simulink model "ANN_MLP_BP_Incremental_Mode_Training"  (Simulink 6.0)
settings: Solver=FixedStepDiscrete  StartTime=0.0  StopTime=10000  RelTol=1e-3
undefined symbols (not defined in the file): magnitude
libraries: simulink x10
settings Model: Creator=marcelo  LastModifiedBy=Marcelo
settings HardwareCC: TargetHWDeviceType=32-bit Generic

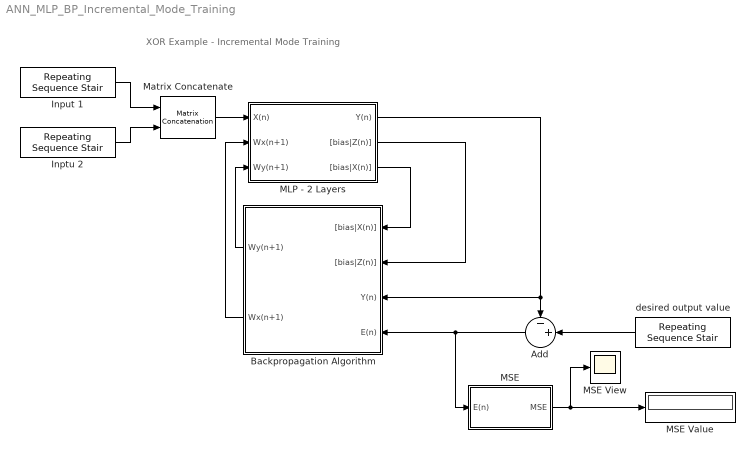
== system ANN_MLP_BP_Incremental_Mode_Training ==
  note: XOR Example - Incremental Mode Training
  Add : Sum  Orientation=left  Inputs=-+|  OutDataType=fixdt(1,16,0)  OutScaling=[]
  Backpropagation Algorithm : Subsystem  Orientation=left  mask(Backpropagation Algorithm){mu=0.2, alpha=0.001, N=1, p=2, H=4, m=1}
      mask prompts: N "training size:"; p "Number of the inputs:"; H "Number of hidden neurons:"; m "Number of output neurons:"
      mask help:
      | Backpropagation Algorithm
      |
      | Prof. Marcelo A. C. Fernandes
      | DCA - CT - UFRN
      | mfernandes@dca.ufrn.br
      mask Help:
      | Backpropagation Algorithm
      | 
      | Prof. Marcelo A. C. Fernandes
      | DCA - CT - UFRN
      | mfernandes@dca.ufrn.br
  Inptu 2 : simulink/Sources/Repeating Sequence Stair  OutValues=[0 1 0 1]  tsamp=1  OutputDataTypeScalingMode=Specify via dialog  OutDataType=float('double')  ConRadixGroup=Best Precision: Vector-wise  OutScaling=2^-12
  Input 1 : simulink/Sources/Repeating Sequence Stair  OutValues=[0 0 1 1]  tsamp=1  OutputDataTypeScalingMode=Specify via dialog  OutDataType=float('double')  ConRadixGroup=Best Precision: Vector-wise  OutScaling=2^-12
  MLP - 2 Layers : Subsystem  mask(Multilayer Perceptron (MLP) - 2 Layers){N=1, valorLimiar=-1, p=2, H=4, m=1}
      mask prompts: N "training size:"; valorLimiar "Bias value:"; p "Number of the inputs:"; H "Number of hidden neurons:"; m "Number of output neurons:"
      mask help:
      | Multilayer Perceptron (MLP) - 2 Layers
      |
      | Prof. Marcelo Augusto Costa Fernandes
      | DCA - CT - UFRN
      | mfernandes@dca.ufrn.br
      mask Help:
      | Multilayer Perceptron (MLP) - 2 Layers
      | 
      | Prof. Marcelo Augusto Costa Fernandes
      | DCA - CT - UFRN
      | mfernandes@dca.ufrn.br
  MSE : Subsystem  mask(MSE){N=1, m=1}
      mask prompts: N "training size:"; m "Number of output neurons:"
      mask help:
      | MSE
      |
      | Prof. Marcelo Augusto Costa Fernandes
      | DCA - CT - UFRN
      | mfernandes@dca.ufrn.br
      mask Help:
      | MSE
      | 
      | Prof. Marcelo Augusto Costa Fernandes
      | DCA - CT - UFRN
      | mfernandes@dca.ufrn.br
  MSE Value : Display
  MSE View : Scope
      settings: MaxDataPoints=5000000
  Matrix Concatenate : simulink/Math Operations/Matrix Concatenation  numInports=2  catMethod=Vertical
  desired output value : simulink/Sources/Repeating Sequence Stair  Orientation=left  OutValues=[0 1 1 0]  tsamp=1  OutputDataTypeScalingMode=Specify via dialog  OutDataType=float('double')  ConRadixGroup=Best Precision: Vector-wise  OutScaling=2^-12
  wires:
  Add/1 -> Backpropagation Algorithm/4(E(n)), MSE/1(E(n))
  MLP - 2 Layers/2("[bias|Z(n)]") -> Backpropagation Algorithm/2("[bias|Z(n)]")
  Backpropagation Algorithm/2(Wx(n+1)) -> MLP - 2 Layers/2(Wx(n+1))
  Backpropagation Algorithm/1(Wy(n+1)) -> MLP - 2 Layers/3(Wy(n+1))
  MLP - 2 Layers/3("[bias|X(n)]") -> Backpropagation Algorithm/1("[bias|X(n)]")
  Input 1/1 -> Matrix Concatenate/1
  Inptu 2/1 -> Matrix Concatenate/2
  MLP - 2 Layers/1(Y(n)) -> Add/1, Backpropagation Algorithm/3(Y(n))
  Matrix Concatenate/1 -> MLP - 2 Layers/1(X(n))
  desired output value/1 -> Add/2
  MSE/1(MSE) -> MSE Value/1, MSE View/1

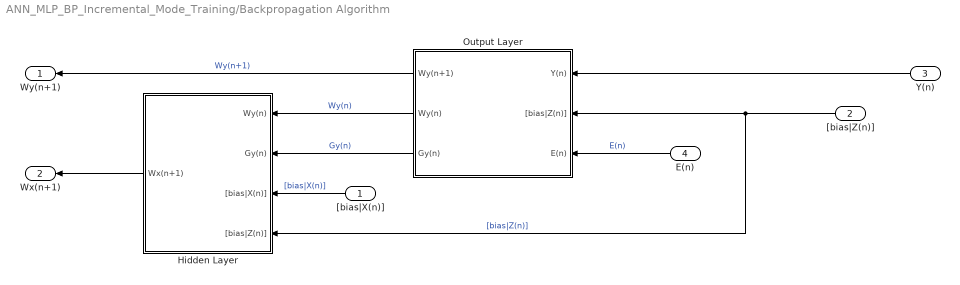
== system ANN_MLP_BP_Incremental_Mode_Training/Backpropagation Algorithm ==
  "[bias|X(n)]" : Inport  Orientation=left  Port=1  OutDataType=fixdt(1,16,0)  OutScaling=[]  LatchInput=off
  "[bias|Z(n)]" : Inport  Orientation=left  Port=2  OutDataType=fixdt(1,16,0)  OutScaling=[]  LatchInput=off
  Y(n) : Inport  Orientation=left  Port=3  OutDataType=fixdt(1,16,0)  OutScaling=[]  LatchInput=off
  E(n) : Inport  Orientation=left  Port=4  OutDataType=fixdt(1,16,0)  OutScaling=[]  LatchInput=off
  Hidden Layer : Subsystem  Orientation=left
  Output Layer : Subsystem  Orientation=left
  Wy(n+1) : Outport  Orientation=left  OutDataType=fixdt(1,16,0)  OutScaling=[]
  Wx(n+1) : Outport  Orientation=left  Port=2  OutDataType=fixdt(1,16,0)  OutScaling=[]
  wires:
  Output Layer/1(Wy(n+1)) -> Wy(n+1)/1  "Wy(n+1)"
  "[bias|Z(n)]"/1 -> Output Layer/2("[bias|Z(n)]"), Hidden Layer/4("[bias|Z(n)]")  "[bias|Z(n)]"
  E(n)/1 -> Output Layer/3(E(n))  "E(n)"
  Output Layer/2(Wy(n)) -> Hidden Layer/1(Wy(n))  "Wy(n)"
  Output Layer/3(Gy(n)) -> Hidden Layer/2(Gy(n))  "Gy(n)"
  "[bias|X(n)]"/1 -> Hidden Layer/3("[bias|X(n)]")  "[bias|X(n)]"
  Hidden Layer/1(Wx(n+1)) -> Wx(n+1)/1
  Y(n)/1 -> Output Layer/1(Y(n))

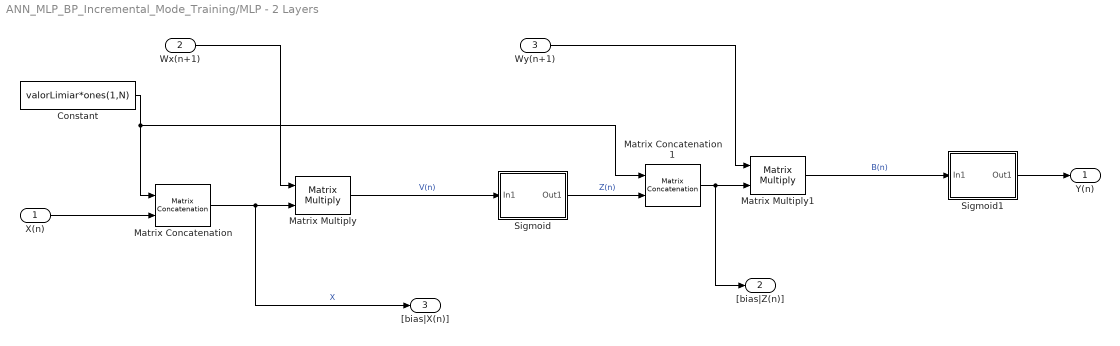
== system ANN_MLP_BP_Incremental_Mode_Training/MLP - 2 Layers ==
  X(n) : Inport  Port=1  OutDataType=fixdt(1,16,0)  OutScaling=[]  LatchInput=off
  Wx(n+1) : Inport  Port=2  OutDataType=fixdt(1,16,0)  OutScaling=[]  LatchInput=off
  Wy(n+1) : Inport  Port=3  OutDataType=fixdt(1,16,0)  OutScaling=[]  LatchInput=off
  Constant : Constant  Value=valorLimiar*ones(1,N)  VectorParams1D=off  OutDataType=fixdt(1,16,0)  OutScaling=[]
  Matrix Concatenation : simulink/Math Operations/Matrix Concatenation  numInports=2  catMethod=Vertical
  Matrix Concatenation1 : simulink/Math Operations/Matrix Concatenation  numInports=2  catMethod=Vertical
  Matrix Multiply : Product  Multiplication=Matrix(*)  OutDataType=fixdt(1,16,0)  OutScaling=[]
  Matrix Multiply1 : Product  Multiplication=Matrix(*)  OutDataType=fixdt(1,16,0)  OutScaling=[]
  Sigmoid : Subsystem
      mask Type: Sigmoid Function
      mask Description:
      | Sigmoid Function.
      | 
      | 1/(1+exp(-x))
      | 
      | Prof. Marcelo Fernandes
      | DCA - CT - UFRN
      | mfernandes@dca.ufrn.br
      mask Help:
      | Sigmoid Function.
      | 
      | 1/(1+exp(-x))
      | 
      | Prof. Marcelo Fernandes
      | DCA - CT - UFRN
      | mfernandes@dca.ufrn.br
      mask Display: plot([-8:.1:8],(1-exp(-1*[-8:.1:8]))./(1+exp(-1*[-8:.1:8])))
  Sigmoid1 : Subsystem
      mask Type: Sigmoid Function
      mask Description:
      | Sigmoid Function.
      | 
      | 1/(1+exp(-x))
      | 
      | Prof. Marcelo Fernandes
      | DCA - CT - UFRN
      | mfernandes@dca.ufrn.br
      mask Help:
      | Sigmoid Function.
      | 
      | 1/(1+exp(-x))
      | 
      | Prof. Marcelo Fernandes
      | DCA - CT - UFRN
      | mfernandes@dca.ufrn.br
      mask Display: plot([-8:.1:8],(1-exp(-1*[-8:.1:8]))./(1+exp(-1*[-8:.1:8])))
  Y(n) : Outport  OutDataType=fixdt(1,16,0)  OutScaling=[]
  "[bias|Z(n)]" : Outport  Port=2  OutDataType=fixdt(1,16,0)  OutScaling=[]
  "[bias|X(n)]" : Outport  Port=3  OutDataType=fixdt(1,16,0)  OutScaling=[]
  wires:
  Constant/1 -> Matrix Concatenation/1, Matrix Concatenation1/1
  Matrix Concatenation/1 -> Matrix Multiply/2, "[bias|X(n)]"/1  "X"
  Matrix Multiply/1 -> Sigmoid/1(In1)  "V(n)"
  X(n)/1 -> Matrix Concatenation/2
  Wx(n+1)/1 -> Matrix Multiply/1
  Matrix Multiply1/1 -> Sigmoid1/1(In1)  "B(n)"
  Sigmoid/1(Out1) -> Matrix Concatenation1/2  "Z(n)"
  Matrix Concatenation1/1 -> Matrix Multiply1/2, "[bias|Z(n)]"/1
  Wy(n+1)/1 -> Matrix Multiply1/1
  Sigmoid1/1(Out1) -> Y(n)/1

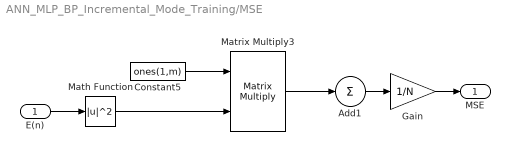
== system ANN_MLP_BP_Incremental_Mode_Training/MSE ==
  E(n) : Inport  Port=1  LatchInput=off
  Add1 : Sum  Inputs=1  OutDataType=fixdt(1,16,0)  OutScaling=[]
  Constant5 : Constant  Value=ones(1,m)  VectorParams1D=off  OutDataType=fixdt(1,16,0)  OutScaling=[]
  Gain : Gain  Gain=1/N  ParameterDataType=fixdt(1,16,0)  ParameterScaling=[]  OutDataType=fixdt(1,16,0)  OutScaling=[]
  Math Function : Math  Operator=magnitude^2  OutDataType=fixdt(1,16,0)  OutScaling=[]  SaturateOnIntegerOverflow=on
  Matrix Multiply3 : Product  Multiplication=Matrix(*)  OutDataType=fixdt(1,16,0)  OutScaling=[]
  MSE : Outport
  wires:
  Add1/1 -> Gain/1
  Constant5/1 -> Matrix Multiply3/1
  Math Function/1 -> Matrix Multiply3/2
  Matrix Multiply3/1 -> Add1/1
  E(n)/1 -> Math Function/1
  Gain/1 -> MSE/1

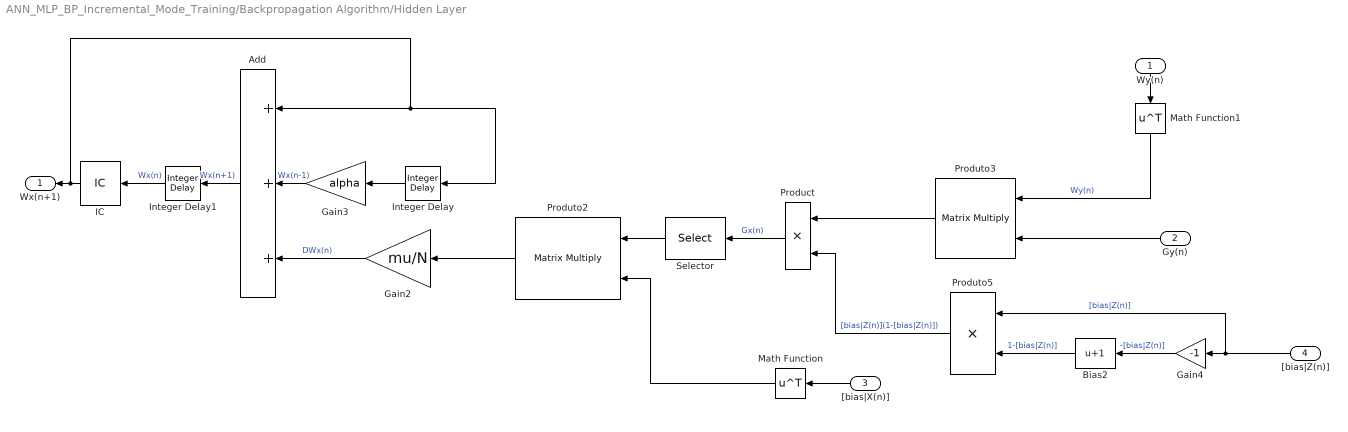
== system ANN_MLP_BP_Incremental_Mode_Training/Backpropagation Algorithm/Hidden Layer ==
  Wy(n) : Inport  Orientation=down  Port=1  OutDataType=fixdt(1,16,0)  OutScaling=[]  LatchInput=off
  Gy(n) : Inport  Orientation=left  Port=2  OutDataType=fixdt(1,16,0)  OutScaling=[]  LatchInput=off
  "[bias|X(n)]" : Inport  Orientation=left  Port=3  OutDataType=fixdt(1,16,0)  OutScaling=[]  LatchInput=off
  "[bias|Z(n)]" : Inport  Orientation=left  Port=4  OutDataType=fixdt(1,16,0)  OutScaling=[]  LatchInput=off
  Add : Sum  Orientation=left  Inputs=+++  OutDataType=fixdt(1,16,0)  OutScaling=[]
  Bias2 : Bias  Orientation=left  Bias=1
  Gain2 : Gain  Orientation=left  Gain=mu/N  ParameterDataType=fixdt(1,16,0)  ParameterScaling=[]  OutDataType=fixdt(1,16,0)  OutScaling=[]
  Gain3 : Gain  Orientation=left  Gain=alpha  ParameterDataType=fixdt(1,16,0)  ParameterScaling=[]  OutDataType=fixdt(1,16,0)  OutScaling=[]
  Gain4 : Gain  Orientation=left  Gain=-1  ParameterDataType=fixdt(1,16,0)  ParameterScaling=[]  OutDataType=fixdt(1,16,0)  OutScaling=[]
  IC : InitialCondition  Orientation=left  Value=rand(H,p+1)
  Integer Delay : simulink/Discrete/Integer Delay  Orientation=left  vinit=0.0  samptime=-1  NumDelays=1
  Integer Delay1 : simulink/Discrete/Integer Delay  Orientation=left  vinit=0.0  samptime=-1  NumDelays=1
  Math Function : Math  Orientation=left  Operator=transpose  OutDataType=fixdt(1,16,0)  OutScaling=[]  SaturateOnIntegerOverflow=on
  Math Function1 : Math  Orientation=down  Operator=transpose  OutDataType=fixdt(1,16,0)  OutScaling=[]  SaturateOnIntegerOverflow=on
  Product : Product  Orientation=left  RndMeth=Zero
  Produto2 : Product  Orientation=left  Inputs=**  Multiplication=Matrix(*)  OutDataType=fixdt(1,16,0)  OutScaling=[]
  Produto3 : Product  Orientation=left  Inputs=**  Multiplication=Matrix(*)  OutDataType=fixdt(1,16,0)  OutScaling=[]
  Produto5 : Product  Orientation=left  Inputs=**  OutDataType=fixdt(1,16,0)  OutScaling=[]
  Selector : Selector  Orientation=left  InputType=Matrix  Rows=[2:H+1]  Columns=-1  InputPortWidth=3
  Wx(n+1) : Outport  Orientation=left  OutDataType=fixdt(1,16,0)  OutScaling=[]
  wires:
  Math Function1/1 -> Produto3/1  "Wy(n)"
  Produto3/1 -> Product/1
  Wy(n)/1 -> Math Function1/1
  Gy(n)/1 -> Produto3/2
  "[bias|X(n)]"/1 -> Math Function/1
  "[bias|Z(n)]"/1 -> Produto5/1, Gain4/1  "[bias|Z(n)]"
  Gain4/1 -> Bias2/1  "-[bias|Z(n)]"
  Bias2/1 -> Produto5/2  "1-[bias|Z(n)]"
  Produto5/1 -> Product/2  "[bias|Z(n)](1-[bias|Z(n)])"
  Product/1 -> Selector/1  "Gx(n)"
  Math Function/1 -> Produto2/2
  Selector/1 -> Produto2/1
  Gain2/1 -> Add/3  "DWx(n)"
  Integer Delay/1 -> Gain3/1
  Gain3/1 -> Add/2  "Wx(n-1)"
  Produto2/1 -> Gain2/1
  Add/1 -> Integer Delay1/1  "Wx(n+1)"
  Integer Delay1/1 -> IC/1  "Wx(n)"
  IC/1 -> Wx(n+1)/1, Add/1, Integer Delay/1

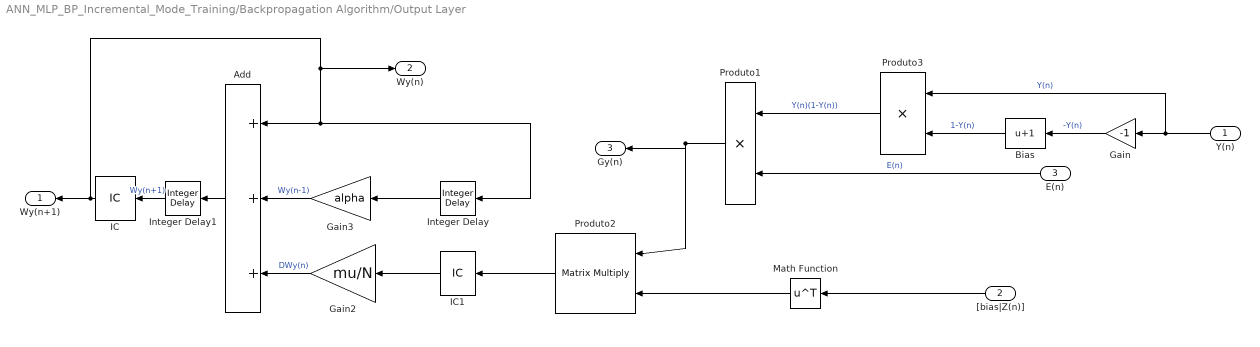
== system ANN_MLP_BP_Incremental_Mode_Training/Backpropagation Algorithm/Output Layer ==
  Y(n) : Inport  Orientation=left  Port=1  OutDataType=fixdt(1,16,0)  OutScaling=[]  LatchInput=off
  "[bias|Z(n)]" : Inport  Orientation=left  Port=2  OutDataType=fixdt(1,16,0)  OutScaling=[]  LatchInput=off
  E(n) : Inport  Orientation=left  Port=3  OutDataType=fixdt(1,16,0)  OutScaling=[]  LatchInput=off
  Add : Sum  Orientation=left  Inputs=+++  OutDataType=fixdt(1,16,0)  OutScaling=[]
  Bias : Bias  Orientation=left  Bias=1
  Gain : Gain  Orientation=left  Gain=-1  ParameterDataType=fixdt(1,16,0)  ParameterScaling=[]  OutDataType=fixdt(1,16,0)  OutScaling=[]
  Gain2 : Gain  Orientation=left  Gain=mu/N  ParameterDataType=fixdt(1,16,0)  ParameterScaling=[]  OutDataType=fixdt(1,16,0)  OutScaling=[]
  Gain3 : Gain  Orientation=left  Gain=alpha  ParameterDataType=fixdt(1,16,0)  ParameterScaling=[]  OutDataType=fixdt(1,16,0)  OutScaling=[]
  IC : InitialCondition  Orientation=left  Value=rand(m,H+1)
  IC1 : InitialCondition  Orientation=left  Value=rand(m,H+1)
  Integer Delay : simulink/Discrete/Integer Delay  Orientation=left  vinit=0.0  samptime=-1  NumDelays=1
  Integer Delay1 : simulink/Discrete/Integer Delay  Orientation=left  vinit=0.0  samptime=-1  NumDelays=1
  Math Function : Math  Orientation=left  Operator=transpose  OutDataType=fixdt(1,16,0)  OutScaling=[]  SaturateOnIntegerOverflow=on
  Produto1 : Product  Orientation=left  Inputs=**  OutDataType=fixdt(1,16,0)  OutScaling=[]
  Produto2 : Product  Orientation=left  Inputs=**  Multiplication=Matrix(*)  OutDataType=fixdt(1,16,0)  OutScaling=[]
  Produto3 : Product  Orientation=left  Inputs=**  OutDataType=fixdt(1,16,0)  OutScaling=[]
  Wy(n+1) : Outport  Orientation=left  OutDataType=fixdt(1,16,0)  OutScaling=[]
  Wy(n) : Outport  Port=2  OutDataType=fixdt(1,16,0)  OutScaling=[]
  Gy(n) : Outport  Orientation=left  Port=3  OutDataType=fixdt(1,16,0)  OutScaling=[]
  wires:
  "[bias|Z(n)]"/1 -> Math Function/1
  Math Function/1 -> Produto2/2
  Gain2/1 -> Add/3  "DWy(n)"
  Integer Delay/1 -> Gain3/1
  Add/1 -> Integer Delay1/1
  Gain3/1 -> Add/2  "Wy(n-1)"
  Integer Delay1/1 -> IC/1  "Wy(n+1)"
  IC/1 -> Wy(n+1)/1, Add/1, Integer Delay/1, Wy(n)/1
  Produto2/1 -> IC1/1
  IC1/1 -> Gain2/1
  E(n)/1 -> Produto1/2  "E(n)"
  Gain/1 -> Bias/1  "-Y(n)"
  Bias/1 -> Produto3/2  "1-Y(n)"
  Produto3/1 -> Produto1/1  "Y(n)(1-Y(n))"
  Produto1/1 -> Produto2/1, Gy(n)/1
  Y(n)/1 -> Gain/1, Produto3/1  "Y(n)"

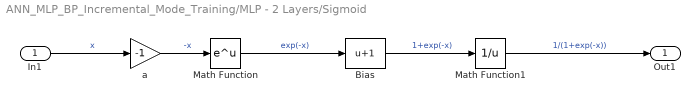
== system ANN_MLP_BP_Incremental_Mode_Training/MLP - 2 Layers/Sigmoid ==
  In1 : Inport  Port=1  OutDataType=fixdt(1,16,0)  OutScaling=[]  LatchInput=off
  Bias : Bias  Bias=1
  Math Function : Math  OutDataType=fixdt(1,16,0)  OutScaling=[]  SaturateOnIntegerOverflow=on
  Math Function1 : Math  Operator=reciprocal  OutDataType=fixdt(1,16,0)  OutScaling=[]  SaturateOnIntegerOverflow=on
  a : Gain  Gain=-1  ParameterDataType=fixdt(1,16,0)  ParameterScaling=[]  OutDataType=fixdt(1,16,0)  OutScaling=[]
  Out1 : Outport  OutDataType=fixdt(1,16,0)  OutScaling=[]
  wires:
  In1/1 -> a/1  "x"
  a/1 -> Math Function/1  "-x"
  Math Function/1 -> Bias/1  "exp(-x)"
  Bias/1 -> Math Function1/1  "1+exp(-x)"
  Math Function1/1 -> Out1/1  "1/(1+exp(-x))"

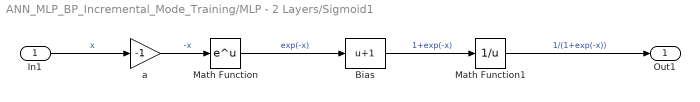
== system ANN_MLP_BP_Incremental_Mode_Training/MLP - 2 Layers/Sigmoid1 ==
  In1 : Inport  Port=1  OutDataType=fixdt(1,16,0)  OutScaling=[]  LatchInput=off
  Bias : Bias  Bias=1
  Math Function : Math  OutDataType=fixdt(1,16,0)  OutScaling=[]  SaturateOnIntegerOverflow=on
  Math Function1 : Math  Operator=reciprocal  OutDataType=fixdt(1,16,0)  OutScaling=[]  SaturateOnIntegerOverflow=on
  a : Gain  Gain=-1  ParameterDataType=fixdt(1,16,0)  ParameterScaling=[]  OutDataType=fixdt(1,16,0)  OutScaling=[]
  Out1 : Outport  OutDataType=fixdt(1,16,0)  OutScaling=[]
  wires:
  Math Function1/1 -> Out1/1  "1/(1+exp(-x))"
  Bias/1 -> Math Function1/1  "1+exp(-x)"
  Math Function/1 -> Bias/1  "exp(-x)"
  a/1 -> Math Function/1  "-x"
  In1/1 -> a/1  "x"
